simulink model "mult2"  (R2016a)
settings: Solver=FixedStepDiscrete  StartTime=0.0  StopTime=10.0  RelTol=1e-3
libraries: rvs x11
settings Model: Creator=Arthur  LastModifiedBy=aeagr
settings DataIOCC: LimitDataPoints=on  SaveFormat=Array
settings DebuggingCC: SolverPrmCheckMsg=warning
settings HardwareCC: ProdBitPerPointer=32  ProdLargestAtomicFloat=None  ProdIntDivRoundTo=Undefined  ProdEndianess=Unspecified  ProdWordSize=32  ProdHWDeviceType=32-bit Generic
settings ModelReferenceCC: PropagateSignalLabelsOutOfModel=off
settings ConfigComp: CovModelRefEnable=Off  CovSFcnEnable=off

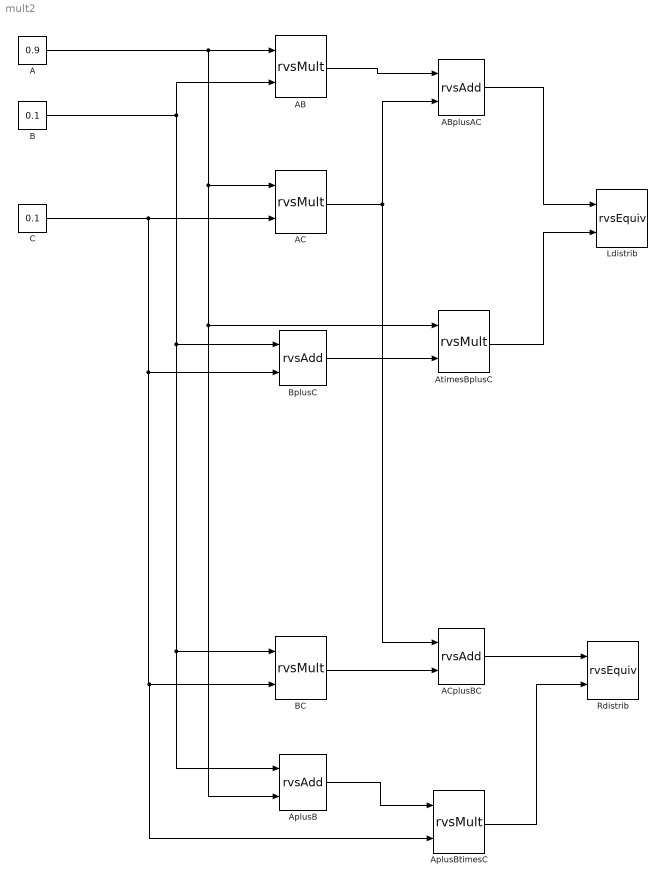
== system mult2 ==
  A : Constant  Value=0.9
  AB : rvs/rvsMult
  ABplusAC : rvs/rvsAdd
  AC : rvs/rvsMult
  ACplusBC : rvs/rvsAdd
  AplusB : rvs/rvsAdd
  AplusBtimesC : rvs/rvsMult
  AtimesBplusC : rvs/rvsMult
  B : Constant  Value=0.1
  BC : rvs/rvsMult
  BplusC : rvs/rvsAdd
  C : Constant  Value=0.1
  Ldistrib : rvs/rvsEquiv  tol=1e-9
  Rdistrib : rvs/rvsEquiv  tol=1e-9
  wires:
  B/1 -> AB/2, AplusB/1, BC/1, BplusC/1
  C/1 -> AplusBtimesC/2, BC/2, BplusC/2, AC/2
  ABplusAC/1 -> Ldistrib/1
  AtimesBplusC/1 -> Ldistrib/2
  A/1 -> AplusB/2, AtimesBplusC/1, AC/1, AB/1
  AB/1 -> ABplusAC/1
  AC/1 -> ACplusBC/1, ABplusAC/2
  BplusC/1 -> AtimesBplusC/2
  BC/1 -> ACplusBC/2
  AplusB/1 -> AplusBtimesC/1
  ACplusBC/1 -> Rdistrib/1
  AplusBtimesC/1 -> Rdistrib/2
